simulink model "q4_c_simulink_PD"  (R2013a)
settings: Solver=ode45  StartTime=0.0  StopTime=10.0  RelTol=1e-3
values from neighbouring files (symbols this model uses):
  Kd = Kd_temp    [f.m]    (also in q4_c_PD.m = x1)
  Kp = Kp_temp    [f.m]    (also in q4_c_PD.m = x2)
settings Model: Creator=obrien94  LastModifiedBy=obrien94

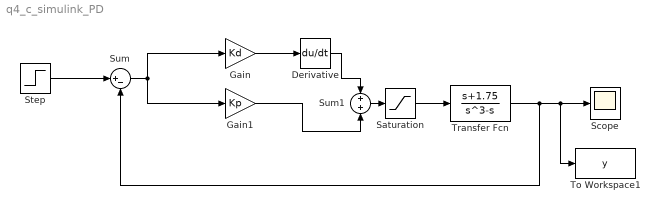
== system q4_c_simulink_PD ==
  Derivative : Derivative
  Gain : Gain  Gain=Kd
  Gain1 : Gain  Gain=Kp
  Saturation : Saturate  UpperLimit=5  LowerLimit=-5
  Scope : Scope
  Step : Step  SampleTime=0
  Sum : Sum  Inputs=|+-
  Sum1 : Sum
  To Workspace1 : ToWorkspace  VariableName=y  SampleTime=-1  SaveFormat=Timeseries
  Transfer Fcn : TransferFcn  Numerator=[1 1.75]  Denominator=[1 0 -1 0]
  wires:
  Step/1 -> Sum/1
  Gain/1 -> Derivative/1
  Derivative/1 -> Sum1/1
  Gain1/1 -> Sum1/2
  Transfer Fcn/1 -> Sum/2, To Workspace1/1, Scope/1
  Sum/1 -> Gain/1, Gain1/1
  Sum1/1 -> Saturation/1
  Saturation/1 -> Transfer Fcn/1
